simulink model "as1_ip_invertedpendulum"  (R2016b)
settings: Solver=FixedStepAuto  StartTime=0.0  StopTime=20  FixedStep=0.001  RelTol=1e-3  EnableMultiTasking=on
values from neighbouring files (symbols this model uses):
  Gd = 60    [as1_ip_run.m]
  Gp = 600    [as1_ip_run.m]
  TD = TDArray(iPar)    [as1_ip_run.m]
libraries: cstblocks x1
settings Model: Creator=KUCKA  LastModifiedBy=cpabl
settings DataIOCC: SaveFormat=Array  ReturnWorkspaceOutputs=on  ReturnWorkspaceOutputsName=yout
settings OptimizationCC: LifeSpan=inf
settings DebuggingCC: UnderspecifiedInitializationDetection=Classic  MergeDetectMultiDrivingBlocksExec=none  SolverPrmCheckMsg=warning  AllowSymbolicDim=off  StateNameClashWarn=warning  SFUnexpectedBacktrackingDiag=warning  SFNoUnconditionalDefaultTransitionDiag=warning  SFExecutionAtInitializationDiag=none
settings HardwareCC: ProdBitPerPointer=32  ProdBitPerSizeT=32  ProdBitPerPtrDiffT=32  ProdLargestAtomicFloat=None  ProdIntDivRoundTo=Undefined  ProdEndianess=Unspecified  ProdWordSize=32  ProdHWDeviceType=32-bit Generic
settings ModelReferenceCC: PropagateSignalLabelsOutOfModel=off
settings GRTTargetCC: TargetLangStandard=C89/C90 (ANSI)  GeneratePreprocessorConditionals=Disable all
settings ConfigComp: CovMetricSettings=dw  CovHtmlReporting=on  CovSaveCumulativeToWorkspaceVar=on  CovSaveSingleToWorkspaceVar=on  CovExternalEMLEnable=off  CovSFcnEnable=off

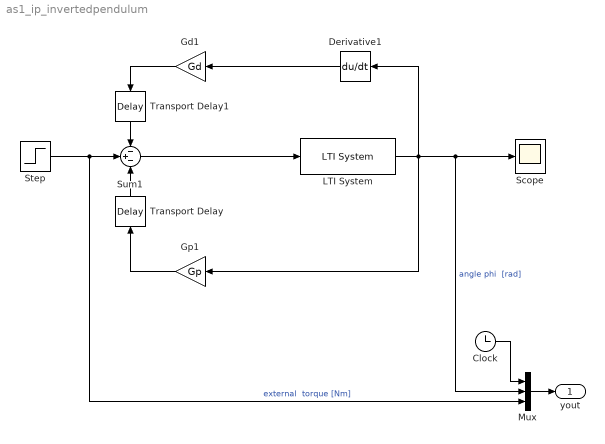
== system as1_ip_invertedpendulum ==
  Clock : Clock
  Derivative1 : Derivative
  Gd1 : Gain  Gain=Gd
  Gp1 : Gain  Gain=Gp
  LTI System : cstblocks/LTI System  sys=H  IC=[]
  Mux : Mux  Inputs=3
  Scope : Scope
  Step : Step  After=5  SampleTime=0
  Sum1 : Sum  Inputs=-+-
  Transport Delay : TransportDelay  DelayTime=TD
  Transport Delay1 : TransportDelay  DelayTime=TD
  yout : Outport
  wires:
  Step/1 -> Sum1/2, Mux/3  "external  torque [Nm]"
  LTI System/1 -> Gp1/1, Derivative1/1, Mux/2, Scope/1  "angle phi  [rad]"
  Mux/1 -> yout/1
  Clock/1 -> Mux/1
  Derivative1/1 -> Gd1/1
  Gd1/1 -> Transport Delay1/1
  Gp1/1 -> Transport Delay/1
  Transport Delay1/1 -> Sum1/1
  Sum1/1 -> LTI System/1
  Transport Delay/1 -> Sum1/3
